simulink model "integrator"  (R2015b)
settings: Solver=VariableStepAuto  StartTime=0.0  StopTime=1  RelTol=1e-3
settings Model: Creator=yehuohanxing  LastModifiedBy=yehuohanxing

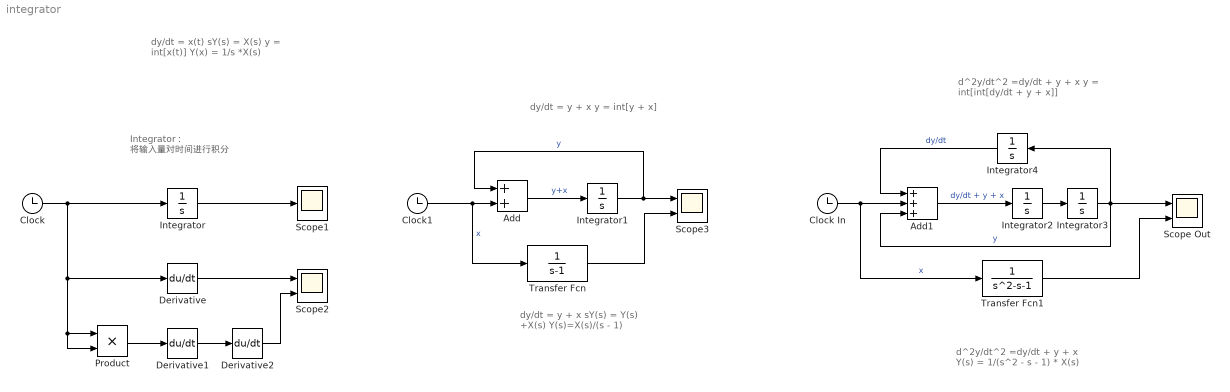
== system integrator ==
  note: dy/dt = y + x
      | y = int[y + x]
  note: dy/dt = x(t)
      | sY(s) = X(s)
      |
      | y = int[x(t)]
      | Y(x) = 1/s *X(s)
  note: Integrator：
      | 将输入量对时间进行积分
  note: dy/dt = y + x
      | sY(s) = Y(s) +X(s)
      | Y(s)=X(s)/(s - 1)
  note: d^2y/dt^2 =dy/dt + y + x
      | y = int[int[dy/dt + y + x]]
  note: d^2y/dt^2 =dy/dt + y + x
      | Y(s) = 1/(s^2 - s - 1) * X(s)
  Add : Sum
  Add1 : Sum  Inputs=+++
  Clock : Clock
  Clock In : Clock
  Clock1 : Clock
  Derivative : Derivative
  Derivative1 : Derivative
  Derivative2 : Derivative
  Integrator{,1..4} (5 alike) : Integrator
  Product : Product
  Scope Out : Scope  NumInputPorts=2
  Scope1 : Scope
  Scope2 : Scope  NumInputPorts=2
  Scope3 : Scope  NumInputPorts=2
  Transfer Fcn : TransferFcn  Denominator=[1 -1]
  Transfer Fcn1 : TransferFcn  Denominator=[1 -1 -1]
  wires:
  Product/1 -> Derivative1/1
  Derivative1/1 -> Derivative2/1
  Clock/1 -> Integrator/1, Derivative/1, Product/2, Product/1
  Derivative2/1 -> Scope2/2
  Clock1/1 -> Transfer Fcn/1, Add/2  "x"
  Add/1 -> Integrator1/1  "y+x"
  Integrator1/1 -> Scope3/1, Add/1  "y"
  Transfer Fcn/1 -> Scope3/2
  Clock In/1 -> Transfer Fcn1/1, Add1/2  "x"
  Add1/1 -> Integrator2/1  "dy/dt + y + x"
  Integrator2/1 -> Integrator3/1
  Integrator3/1 -> Integrator4/1, Add1/3, Scope Out/1  "y"
  Integrator4/1 -> Add1/1  "dy/dt"
  Transfer Fcn1/1 -> Scope Out/2
  Integrator/1 -> Scope1/1
  Derivative/1 -> Scope2/1
